simulink model "auv_modell"  (Simulink 7.1)
settings: Solver=ode45  StartTime=0.0  StopTime=500.0  RelTol=1e-3
libraries: marine_gnc x2, vrlib x1, simulink x1
settings Model: Creator=anderga  LastModifiedBy=anderga

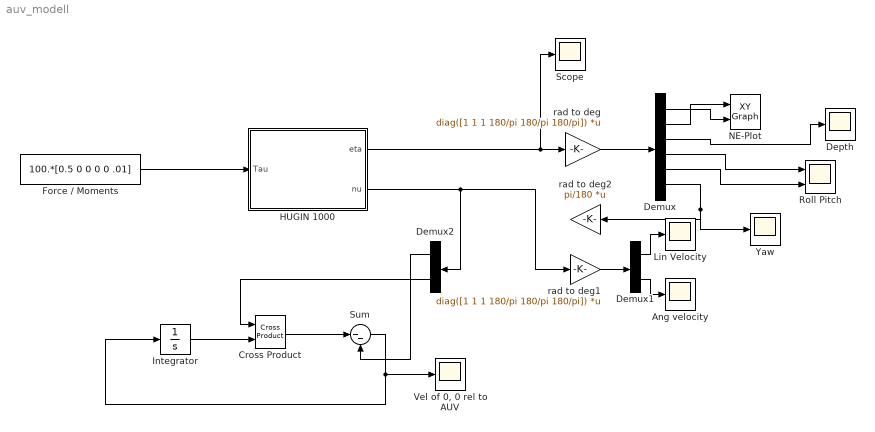
== system auv_modell ==
  Ang velocity : Scope
      settings: YMin=-12  YMax=1  SaveName=ScopeData6
  Cross Product : vrlib/Utilities/Cross Product  SystemSampleTime=-1
  Demux : Demux  Outputs=6
  Demux1 : Demux  Outputs=2
  Demux2 : Demux  Orientation=left  Outputs=2
  Depth : Scope
      settings: YMin=-1  YMax=14  SaveName=ScopeData4
  Force / Moments : Constant  Value=100.*[0.5 0 0 0 0 .01]  OutDataType=sfix(16)  OutScaling=2^0
  HUGIN 1000 : Subsystem  mask{eta_0=[100 100 0 0 0 0], nu_0=[0 0 0 0 0 0], beta_c=0, v_c=0}
      mask prompts: eta_0 "Initial Position [x y z phi theta psi]"; nu_0 "Initial speed [u v w p q r]"; beta_c "Current heading (deg)"; v_c "Current Speed (m/s)"
      mask init:
      | m = 1380;
      | xg = 0;
      | yg = 0;
      | zg = 0.0328;
      | Ix = 86.53;
      | Iy = 1247;
      | Iz = 1247;
      | 
      | M_RB = [m 0 0 0 m*zg -m*yg;
      |         0 m 0 -m*zg 0 m*xg;
      |         0 0 m m*yg -m*xg 0;
      |         0 -m*zg m*yg Ix 0 0;
      |         m*zg 0 -m*xg 0 Iy 0;
      |         -m*yg m*xg 0 0 0 Iz];
      | 
      | Xu = -85.57;
      | Yv = -1092.9;
      | Yr = -84.1448;
      | Zw = -1092.9;
      | Zq = 84.1448;
      | Mq = -795.1686;
      | Nr = -795.1686;
      |     
      | M_A = [-Xu 0 0 0 0 0;
      |         0 -Yv 0 0 0 0;
      |         0 0 -Zw 0 -Zq 0;
      |         0 0 0 0 0 0;
      |         0 0 -Zq 0 -Mq 0;
      |         0 -Yr 0 0 0 -Nr];
  Integrator : Integrator  InitialCondition=[-100 100 0]'
  Lin Velocity : Scope
      settings: YMin=-0.0025  YMax=0.0375
  NE-Plot : simulink/Sinks/XY Graph  SystemSampleTime=-1  xmin=-500  xmax=500  ymin=-500  ymax=500  st=-1
  Roll Pitch : Scope  NumInputPorts=2
      settings: YMin=-0.00125~-1  YMax=0~8  SaveName=ScopeData3
  Scope : Scope
  Sum : Sum  Inputs=|--  OutDataType=sfix(16)  OutScaling=2^0
  "Vel of 0, 0 rel to AUV" : Scope
      settings: YMin=-2  YMax=0.25  SaveName=ScopeData7
  Yaw : Scope
      settings: TimeRange=100  YMin=0.19  YMax=0.24  SaveName=ScopeData2
  rad to deg : Gain  Gain=diag([1 1 1 180/pi 180/pi 180/pi])  Multiplication=Matrix(K*u)  ParameterDataType=sfix(16)  ParameterScaling=2^0  OutDataType=sfix(16)  OutScaling=2^0
  rad to deg1 : Gain  Gain=diag([1 1 1 180/pi 180/pi 180/pi])  Multiplication=Matrix(K*u)  ParameterDataType=sfix(16)  ParameterScaling=2^0  OutDataType=sfix(16)  OutScaling=2^0
  rad to deg2 : Gain  Orientation=left  Gain=pi/180  Multiplication=Matrix(K*u)  ParameterDataType=sfix(16)  ParameterScaling=2^0  OutDataType=sfix(16)  OutScaling=2^0
  wires:
  Force / Moments/1 -> HUGIN 1000/1(Tau)
  HUGIN 1000/1(eta) -> Scope/1, rad to deg/1
  Demux/2 -> NE-Plot/1
  Demux/1 -> NE-Plot/2
  Demux/6 -> Yaw/1, rad to deg2/1
  Demux/4 -> Roll Pitch/1
  Demux/5 -> Roll Pitch/2
  Demux/3 -> Depth/1
  Demux1/1 -> Lin Velocity/1
  Demux1/2 -> Ang velocity/1
  HUGIN 1000/2(nu) -> rad to deg1/1, Demux2/1
  rad to deg/1 -> Demux/1
  rad to deg1/1 -> Demux1/1
  Demux2/1 -> Sum/2
  Integrator/1 -> Cross Product/2
  Demux2/2 -> Cross Product/1
  Cross Product/1 -> Sum/1
  Sum/1 -> "Vel of 0, 0 rel to AUV"/1, Integrator/1

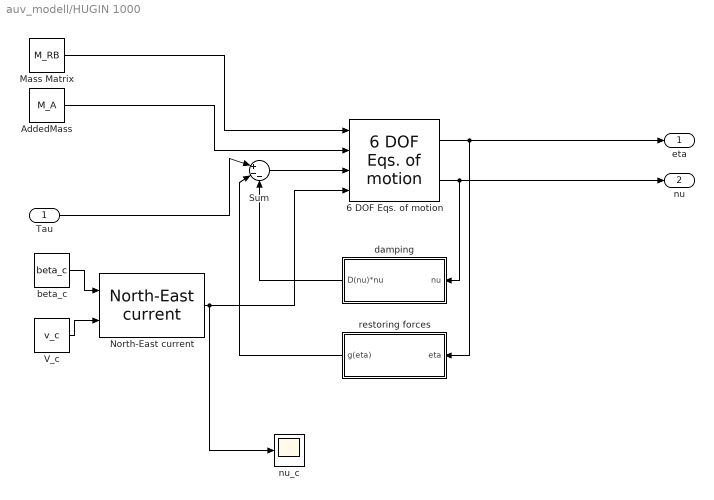
== system auv_modell/HUGIN 1000 ==
  Tau : Inport  OutDataType=sfix(16)  OutScaling=2^0
  " nu_c" : Scope
      settings: TimeRange=100  YMin=0  YMax=1.5  SaveName=ScopeData5
  6 DOF Eqs. of motion : marine_gnc/Models/ Kinetics /6 DOF Eqs. of motion  SystemSampleTime=-1  CoriolisOnOff=on  nu0=nu_0  eta0=eta_0
  AddedMass : Constant  Value=M_A  OutDataType=sfix(16)  OutScaling=2^0
  Mass Matrix : Constant  Value=M_RB  OutDataType=sfix(16)  OutScaling=2^0
  North-East current : marine_gnc/Environment/Current/North-East current  SystemSampleTime=-1
  Sum : Sum  Inputs=|+--  OutDataType=sfix(16)  OutScaling=2^0
  V_c : Constant  Value=v_c  OutDataType=sfix(16)  OutScaling=2^0
  beta_c : Constant  Value=beta_c  OutDataType=sfix(16)  OutScaling=2^0
  damping : Subsystem  Orientation=left
      mask init:
      | Xu = -19.1881;
      | Yv = -931.9715;
      | Yr = 1915.8;
      | Zw = -931.9715;
      | Zq = -1915.8;
      | Kp = -1000;
      | Mw = 1760.7;
      | Mq = -8386.3;
      | Nv = -1760.7;
      | Nr = -8386.3;
      | 
      | Xuu = -3.8938;
      | 
      | D = [Xu 0 0 0 0 0;
      |       0 Yv 0 0 0 Yr;
      |       0 0 Zw 0 Zq 0;
      |       0 0 0 Kp 0 0;
      |       0 0 Mw 0 Mq 0;
      |       0 Nv 0 0 0 Nr];
  restoring forces : Subsystem  Orientation=left
      mask init:
      | W = 1380*9.81;
      | 
      | zg = 0.0328;
  eta : Outport  OutDataType=sfix(16)  OutScaling=2^0
  nu : Outport  Port=2  OutDataType=sfix(16)  OutScaling=2^0
  wires:
  Mass Matrix/1 -> 6 DOF Eqs. of motion/1
  AddedMass/1 -> 6 DOF Eqs. of motion/2
  6 DOF Eqs. of motion/2 -> damping/1(nu), nu/1
  6 DOF Eqs. of motion/1 -> restoring forces/1(eta), eta/1
  restoring forces/1(g(eta)) -> Sum/2
  damping/1(D(nu)*nu) -> Sum/3
  Sum/1 -> 6 DOF Eqs. of motion/3
  Tau/1 -> Sum/1
  North-East current/1 -> 6 DOF Eqs. of motion/4, " nu_c"/1
  beta_c/1 -> North-East current/1
  V_c/1 -> North-East current/2

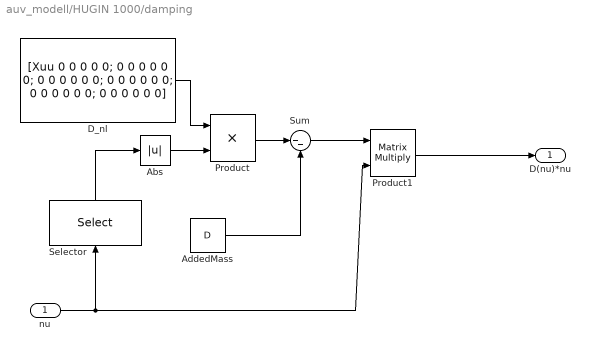
== system auv_modell/HUGIN 1000/damping ==
  nu : Inport  OutDataType=sfix(16)  OutScaling=2^0
  Abs : Abs  OutDataType=sfix(16)  OutScaling=2^0
  AddedMass : Constant  Value=D  OutDataType=sfix(16)  OutScaling=2^0
  D_nl : Constant  Value=[Xuu 0 0 0 0 0; 0 0 0 0 0 0; 0 0 0 0 0 0; 0 0 0 0 0 0; 0 0 0 0 0 0; 0 0 0 0 0 0]  OutDataType=sfix(16)  OutScaling=2^0
  Product : Product  OutDataType=sfix(16)  OutScaling=2^0  RndMeth=Zero
  Product1 : Product  Multiplication=Matrix(*)  OutDataType=sfix(16)  OutScaling=2^0  RndMeth=Zero
  Selector : Selector  Orientation=up  InputPortWidth=6  IndexOptions=Index vector (dialog)  Indices=[1]  OutputSizes=1
  Sum : Sum  Inputs=|--  OutDataType=sfix(16)  OutScaling=2^0
  D(nu)*nu : Outport  OutDataType=sfix(16)  OutScaling=2^0
  wires:
  AddedMass/1 -> Sum/2
  Product/1 -> Sum/1
  nu/1 -> Product1/2, Selector/1
  D_nl/1 -> Product/1
  Abs/1 -> Product/2
  Sum/1 -> Product1/1
  Product1/1 -> D(nu)*nu/1
  Selector/1 -> Abs/1

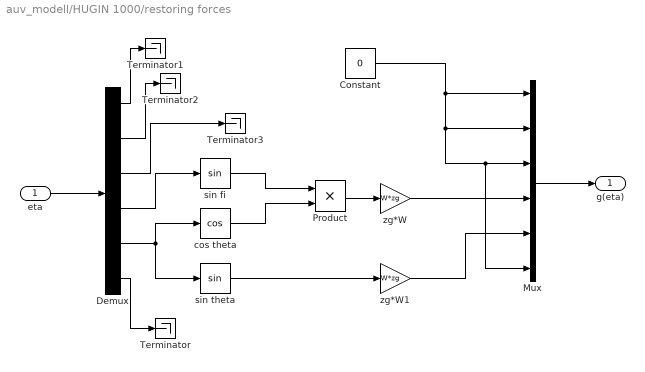
== system auv_modell/HUGIN 1000/restoring forces ==
  eta : Inport  OutDataType=sfix(16)  OutScaling=2^0
  Constant : Constant  Value=0  OutDataType=sfix(16)  OutScaling=2^0
  Demux : Demux  Outputs=6
  Mux : Mux  Inputs=6
  Product : Product  OutDataType=sfix(16)  OutScaling=2^0  RndMeth=Zero
  Terminator{,1..3} (4 alike) : Terminator
  cos theta : Trigonometry  Operator=cos
  sin fi : Trigonometry
  sin theta : Trigonometry
  zg*W : Gain  Gain=W*zg  ParameterDataType=sfix(16)  ParameterScaling=2^0  OutDataType=sfix(16)  OutScaling=2^0
  zg*W1 : Gain  Gain=W*zg  ParameterDataType=sfix(16)  ParameterScaling=2^0  OutDataType=sfix(16)  OutScaling=2^0
  g(eta) : Outport  OutDataType=sfix(16)  OutScaling=2^0
  wires:
  eta/1 -> Demux/1
  Demux/4 -> sin fi/1
  Demux/5 -> cos theta/1, sin theta/1
  cos theta/1 -> Product/2
  sin fi/1 -> Product/1
  Product/1 -> zg*W/1
  sin theta/1 -> zg*W1/1
  Mux/1 -> g(eta)/1
  zg*W1/1 -> Mux/5
  zg*W/1 -> Mux/4
  Constant/1 -> Mux/1, Mux/2, Mux/3, Mux/6
  Demux/6 -> Terminator/1
  Demux/1 -> Terminator1/1
  Demux/2 -> Terminator2/1
  Demux/3 -> Terminator3/1
